simulink library "VEH_CAN"  (R2017a)
settings: Solver=VariableStepAuto  StartTime=0.0  StopTime=10.0  RelTol=1e-3
settings Model: Creator=Di Russo  LastModifiedBy=Vraj M

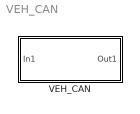
== system VEH_CAN ==
  VEH_CAN : Subsystem

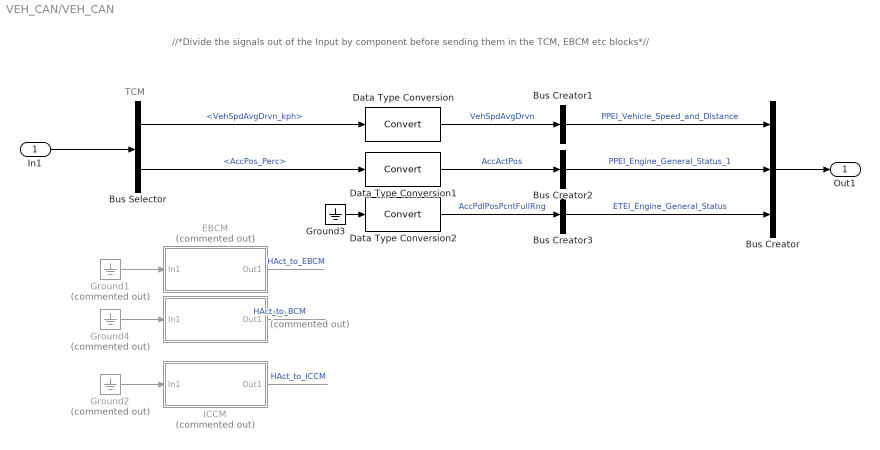
== system VEH_CAN/VEH_CAN ==
  note: //*Divide the signals out of the Input by component before sending them in the TCM, EBCM etc blocks*//
  note: TCM
  In1 : Inport
  BCM : Subsystem  Commented=on
  Bus Creator : BusCreator  Inputs=3
  Bus Creator1 : BusCreator  Inputs=1
  Bus Creator2 : BusCreator  Inputs=1
  Bus Creator3 : BusCreator  Inputs=1
  Bus Selector : BusSelector  OutputSignals=Controls.VehSpdAvgDrvn_kph,Controls.AccPos_Perc
  Data Type Conversion : DataTypeConversion
  Data Type Conversion1 : DataTypeConversion
  Data Type Conversion2 : DataTypeConversion
  EBCM : Subsystem  Commented=on
  Ground1 : Ground  Commented=on
  Ground2 : Ground  Commented=on
  Ground3 : Ground
  Ground4 : Ground  Commented=on
  ICCM : Subsystem  Commented=on
  Out1 : Outport
  wires:
  Ground4/1 -> BCM/1(In1)
  Ground3/1 -> Data Type Conversion2/1
  Data Type Conversion2/1 -> Bus Creator3/1  "AccPdlPosPcntFullRng"
  Bus Creator3/1 -> Bus Creator/3  "ETEI_Engine_General_Status"
  Bus Creator2/1 -> Bus Creator/2  "PPEI_Engine_General_Status_1"
  Data Type Conversion1/1 -> Bus Creator2/1  "AccActPos"
  Bus Creator1/1 -> Bus Creator/1  "PPEI_Vehicle_Speed_and_Distance"
  In1/1 -> Bus Selector/1
  Bus Selector/1 -> Data Type Conversion/1  "<VehSpdAvgDrvn_kph>"
  Bus Selector/2 -> Data Type Conversion1/1  "<AccPos_Perc>"
  Ground2/1 -> ICCM/1(In1)
  Ground1/1 -> EBCM/1(In1)
  Bus Creator/1 -> Out1/1
  Data Type Conversion/1 -> Bus Creator1/1  "VehSpdAvgDrvn"
  EBCM/1(Out1) -> ?  "HAct_to_EBCM"
  BCM/1(Out1) -> ?  "HAct_to_BCM"
  ICCM/1(Out1) -> ?  "HAct_to_ICCM"

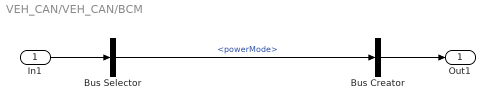
== system VEH_CAN/VEH_CAN/BCM ==
  In1 : Inport
  Bus Creator : BusCreator  Inputs=1
  Bus Selector : BusSelector  OutputSignals=Controls.powerMode
  Out1 : Outport
  wires:
  Bus Creator/1 -> Out1/1
  Bus Selector/1 -> Bus Creator/1  "<powerMode>"
  In1/1 -> Bus Selector/1

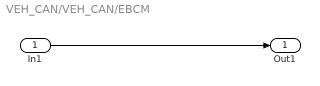
== system VEH_CAN/VEH_CAN/EBCM ==
  In1 : Inport
  Out1 : Outport
  wires:
  In1/1 -> Out1/1

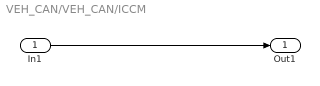
== system VEH_CAN/VEH_CAN/ICCM ==
  In1 : Inport
  Out1 : Outport
  wires:
  In1/1 -> Out1/1
